simulink model "dcm1"  (R2023a)
settings: Solver=ode45  StartTime=0.0  StopTime=2  RelTol=1e-3  EnableMultiTasking=on
undefined symbols (not defined in the file or in its folder): dcm
settings Model: Creator=jkempkes  LastModifiedBy=herranz
settings SolverCC: AlgebraicLoopSolver=TrustRegion
settings DataIOCC: LimitDataPoints=on  SaveFormat=Array  SignalLoggingSaveFormat=ModelDataLogs  ReturnWorkspaceOutputs=off  SignalLoggingName=sigsOut
settings OptimizationCC: BooleanDataType=off  LifeSpan=inf
settings DebuggingCC: SaveWithParameterizedLinksMsg=none  UnderspecifiedInitializationDetection=Classic  MergeDetectMultiDrivingBlocksExec=none  SignalResolutionControl=TryResolveAllWithWarning  MultiTaskDSMMsg=warning  MultiTaskCondExecSysMsg=none  UnconnectedInputMsg=warning  UnconnectedOutputMsg=warning  UnconnectedLineMsg=warning  SFUnexpectedBacktrackingDiag=warning  SFNoUnconditionalDefaultTransitionDiag=warning  SFExecutionAtInitializationDiag=none  ArithmeticOperatorsInVariantConditions=warning
settings HardwareCC: ProdBitPerPointer=32  ProdBitPerSizeT=32  ProdBitPerPtrDiffT=32  ProdLargestAtomicFloat=None  ProdIntDivRoundTo=Undefined  ProdEndianess=Unspecified  ProdWordSize=32  ProdHWDeviceType=32-bit Generic  TargetUnknown=on
settings ModelReferenceCC: PropagateSignalLabelsOutOfModel=off
settings SFSimCC: SimUseLocalCustomCode=off  CustomCodeUndefinedFunction=UseInterfaceOnly
settings RTWCC: RTWUseLocalCustomCode=off
settings CodeAppCC: StateflowObjectComments=on
settings GRTTargetCC: TargetLangStandard=C89/C90 (ANSI)  CombineOutputUpdateFcns=off  GRTInterface=on
settings ConfigComp: CovMetricSettings=dw  CovSaveCumulativeToWorkspaceVar=on  CovSaveSingleToWorkspaceVar=on  CovExternalEMLEnable=off

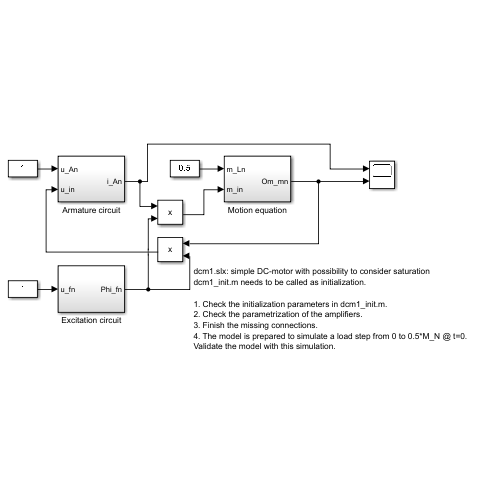
[thumbnail: Simulink's stored preview of the top-level diagram]
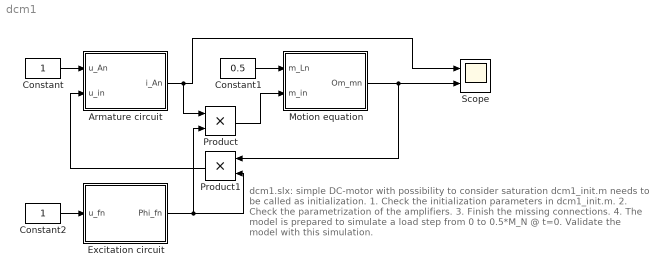
== system dcm1 ==
  note: dcm1.slx: simple DC-motor with possibility to consider saturation
      | dcm1_init.m needs to be called as initialization.
      |
      | 1. Check the initialization parameters in dcm1_init.m.
      | 2. Check the parametrization of the amplifiers.
      | 3. Finish the missing connections.
      | 4. The model is prepared to simulate a load step from 0 to 0.5*M_N @ t=0. Validate the model with this simulation.
  Armature circuit : Subsystem
  Constant : Constant
  Constant1 : Constant  Value=0.5
  Constant2 : Constant
  Excitation circuit : Subsystem
  Motion equation : Subsystem
  Product : Product  InputSameDT=on  SaturateOnIntegerOverflow=on  OutDataTypeStr=Inherit: Same as first input
  Product1 : Product  InputSameDT=on  SaturateOnIntegerOverflow=on  OutDataTypeStr=Inherit: Same as first input
  Scope : Scope  NumInputPorts=2
  wires:
  Constant/1 -> Armature circuit/1(u_An)
  Constant2/1 -> Excitation circuit/1(u_fn)
  Constant1/1 -> Motion equation/1(m_Ln)
  Motion equation/1(Om_mn) -> Product1/1, Scope/2
  Armature circuit/1(i_An) -> Product/1, Scope/1
  Excitation circuit/1(Phi_fn) -> Product/2, Product1/2
  Product1/1 -> Armature circuit/2(u_in)
  Product/1 -> Motion equation/2(m_in)

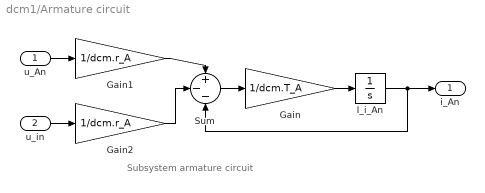
== system dcm1/Armature circuit ==
  note: Subsystem armature circuit
  u_An : Inport
  u_in : Inport  Port=2
  Gain : Gain  Gain=1/dcm.T_A  SaturateOnIntegerOverflow=on  OutDataTypeStr=Inherit: Same as input  ParamDataTypeStr=Inherit: Same as input
  Gain1 : Gain  Gain=1/dcm.r_A  SaturateOnIntegerOverflow=on  OutDataTypeStr=Inherit: Same as input  ParamDataTypeStr=Inherit: Same as input
  Gain2 : Gain  Gain=1/dcm.r_A  SaturateOnIntegerOverflow=on  OutDataTypeStr=Inherit: Same as input  ParamDataTypeStr=Inherit: Same as input
  I_i_An : Integrator
  Sum : Sum  Inputs=+--  InputSameDT=on  SaturateOnIntegerOverflow=on  OutDataTypeStr=Inherit: Same as first input
  i_An : Outport
  wires:
  Gain/1 -> I_i_An/1
  Sum/1 -> Gain/1
  u_An/1 -> Gain1/1
  u_in/1 -> Gain2/1
  Gain1/1 -> Sum/1
  Gain2/1 -> Sum/2
  I_i_An/1 -> Sum/3, i_An/1

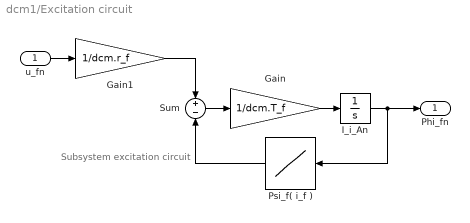
== system dcm1/Excitation circuit ==
  note: Subsystem excitation circuit
  u_fn : Inport
  Gain : Gain  Gain=1/dcm.T_f  SaturateOnIntegerOverflow=on  OutDataTypeStr=Inherit: Same as input  ParamDataTypeStr=Inherit: Same as input
  Gain1 : Gain  Gain=1/dcm.r_f  SaturateOnIntegerOverflow=on  OutDataTypeStr=Inherit: Same as input  ParamDataTypeStr=Inherit: Same as input
  I_i_An : Integrator  InitialCondition=dcm.Pfi_f0
  Psi_f( i_f ) : Lookup  InputValues=dcm.Phi_f  Table=dcm.i_f
  Sum : Sum  Inputs=+-  InputSameDT=on  SaturateOnIntegerOverflow=on  OutDataTypeStr=Inherit: Same as first input
  Phi_fn : Outport
  wires:
  u_fn/1 -> Gain1/1
  I_i_An/1 -> Psi_f( i_f )/1, Phi_fn/1
  Gain/1 -> I_i_An/1
  Sum/1 -> Gain/1
  Gain1/1 -> Sum/1
  Psi_f( i_f )/1 -> Sum/2

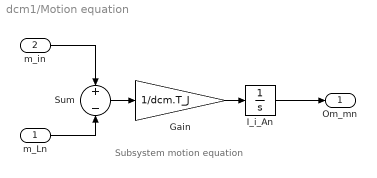
== system dcm1/Motion equation ==
  note: Subsystem motion equation
  m_Ln : Inport
  m_in : Inport  Port=2
  Gain : Gain  Gain=1/dcm.T_J  SaturateOnIntegerOverflow=on  OutDataTypeStr=Inherit: Same as input  ParamDataTypeStr=Inherit: Same as input
  I_i_An : Integrator  InitialCondition=dcm.Om_m0
  Sum : Sum  Inputs=+-  InputSameDT=on  SaturateOnIntegerOverflow=on  OutDataTypeStr=Inherit: Same as first input
  Om_mn : Outport
  wires:
  I_i_An/1 -> Om_mn/1
  Sum/1 -> Gain/1
  Gain/1 -> I_i_An/1
  m_in/1 -> Sum/1
  m_Ln/1 -> Sum/2
